simulink model "GraneBaseModel"  (R2023b)
settings: Solver=ode1  StartTime=0.0  StopTime=10  FixedStep=0.01  RelTol=1e-3
undefined symbols (not defined in the file or in its folder): DiscIntNeverNeededParam, National_Instruments, PCI
libraries: sldrtlib x4, simulink x2
settings Model: Creator=labadmin  LastModifiedBy=labadmin
settings SolverCC: AlgebraicLoopSolver=TrustRegion
settings DataIOCC: ReturnWorkspaceOutputs=off
settings DebuggingCC: UnconnectedInputMsg=warning  UnconnectedOutputMsg=warning  UnconnectedLineMsg=warning  ArithmeticOperatorsInVariantConditions=warning
settings HardwareCC: ProdBitPerLong=64  ProdHWDeviceType=Intel->x86-64 (Linux 64)
settings ModelReferenceCC: EnableRefExpFcnMdlSchedulingChecks=on
settings SFSimCC: SimUseLocalCustomCode=off  CustomCodeUndefinedFunction=UseInterfaceOnly
settings RTWCC: Description=Simulink Desktop Real-Time  SystemTargetFile=sldrt.tlc  TemplateMakefile=sldrt.tmf  RTWUseLocalCustomCode=off  RTWCompilerOptimization=on
settings CodeAppCC: MaxIdLength=95
settings SimulinkDesktopRealTimeCC: TargetLibSuffix=_sldrt.a  TargetPreCompLibLocation=C:\Program Files\MATLAB\R2023b\toolbox\sldrt\lib\win64

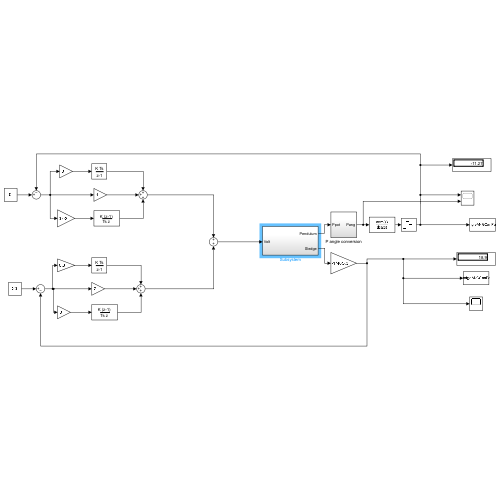
[thumbnail: Simulink's stored preview of the top-level diagram]
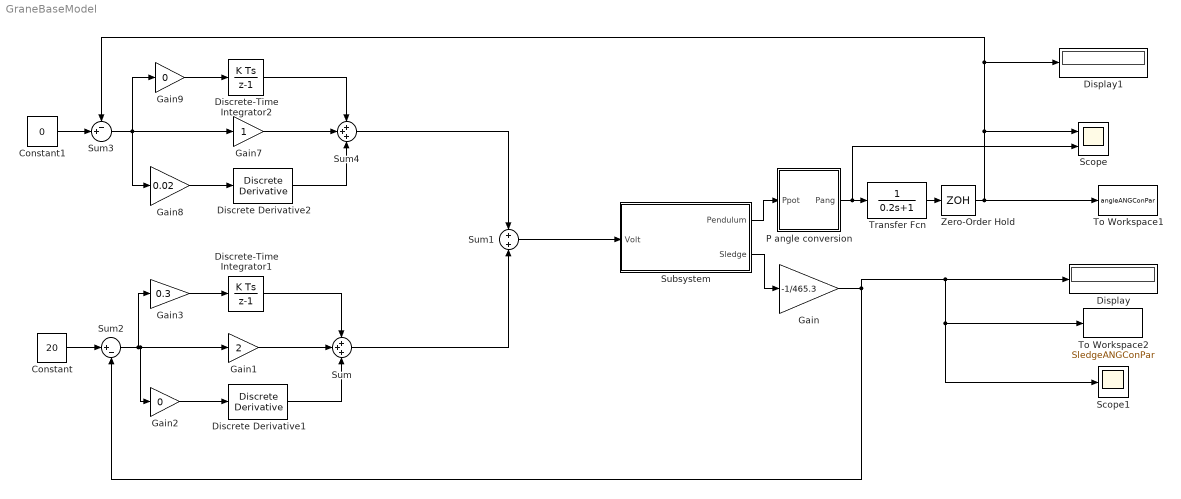
== system GraneBaseModel ==
  Constant : Constant  Value=20
  Constant1 : Constant  Value=0
  Discrete Derivative1 : simulink/Discrete/Discrete Derivative  gainval=1.0  ICPrevScaledInput=0.0  OutMin=[]  OutMax=[]  OutDataType=fixdt(1, 16)  OutScaling=2^-10  DoSatur=off
  Discrete Derivative2 : simulink/Discrete/Discrete Derivative  gainval=1.0  ICPrevScaledInput=0.0  OutMin=[]  OutMax=[]  OutDataType=fixdt(1, 16)  OutScaling=2^-10  DoSatur=off
  Discrete-Time Integrator1 : DiscreteIntegrator  SampleTime=-1  ICPrevOutput=DiscIntNeverNeededParam  ICPrevScaledInput=DiscIntNeverNeededParam
  Discrete-Time Integrator2 : DiscreteIntegrator  SampleTime=-1  ICPrevOutput=DiscIntNeverNeededParam  ICPrevScaledInput=DiscIntNeverNeededParam
  Display : Display
  Display1 : Display
  Gain : Gain  Gain=-1/465.3
  Gain1 : Gain  Gain=2
  Gain2 : Gain  Gain=0
  Gain3 : Gain  Gain=0.3
  Gain7 : Gain
  Gain8 : Gain  Gain=0.02
  Gain9 : Gain  Gain=0
  P angle conversion : Subsystem
  Scope : Scope  NumInputPorts=2
  Scope1 : Scope
  Subsystem : Subsystem
  Sum : Sum  Inputs=+++
  Sum1 : Sum
  Sum2 : Sum  Inputs=|+-
  Sum3 : Sum  Inputs=-+|
  Sum4 : Sum  Inputs=+++
  To Workspace1 : ToWorkspace  VariableName=angleANGConPar  SaveFormat=Timeseries  SampleTime=-1
  To Workspace2 : ToWorkspace  VariableName=SledgeANGConPar  SaveFormat=Timeseries  SampleTime=-1
  Transfer Fcn : TransferFcn  Denominator=[0.2 1]
  Zero-Order Hold : ZeroOrderHold  SampleTime=-1
  wires:
  Subsystem/2(Sledge) -> Gain/1
  Subsystem/1(Pendulum) -> P angle conversion/1(Ppot)
  Gain/1 -> To Workspace2/1, Scope1/1, Display/1, Sum2/2
  Gain1/1 -> Sum/2
  Discrete Derivative1/1 -> Sum/3
  Gain3/1 -> Discrete-Time Integrator1/1
  Gain2/1 -> Discrete Derivative1/1
  Constant/1 -> Sum2/1
  Sum2/1 -> Gain3/1, Gain2/1, Gain1/1
  Discrete-Time Integrator1/1 -> Sum/1
  P angle conversion/1(Pang) -> Scope/2, Transfer Fcn/1
  Zero-Order Hold/1 -> Sum3/1, Display1/1, Scope/1, To Workspace1/1
  Transfer Fcn/1 -> Zero-Order Hold/1
  Gain9/1 -> Discrete-Time Integrator2/1
  Discrete Derivative2/1 -> Sum4/3
  Gain7/1 -> Sum4/2
  Discrete-Time Integrator2/1 -> Sum4/1
  Gain8/1 -> Discrete Derivative2/1
  Sum4/1 -> Sum1/1
  Sum/1 -> Sum1/2
  Constant1/1 -> Sum3/2
  Sum3/1 -> Gain8/1, Gain7/1, Gain9/1
  Sum1/1 -> Subsystem/1(Volt)

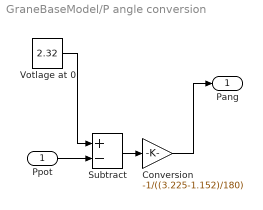
== system GraneBaseModel/P angle conversion ==
  Ppot : Inport
  Conversion : Gain  Gain=-1/((3.225-1.152)/180)
  Subtract : Sum  Inputs=+-
  "Votlage at 0 " : Constant  Value=2.32
  Pang : Outport  VectorParamsAs1DForOutWhenUnconnected=off
  wires:
  Subtract/1 -> Conversion/1
  Ppot/1 -> Subtract/2
  "Votlage at 0 "/1 -> Subtract/1
  Conversion/1 -> Pang/1

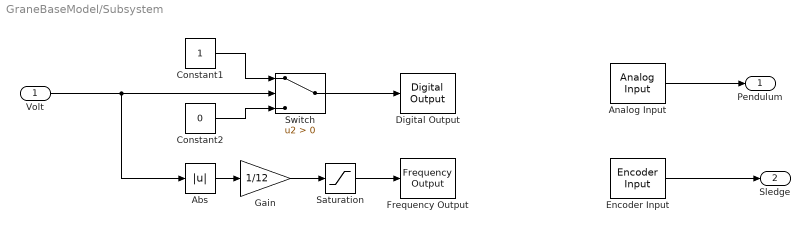
== system GraneBaseModel/Subsystem ==
  Volt : Inport
  Abs : Abs  SaturateOnIntegerOverflow=off
  Analog Input : sldrtlib/Analog Input  SampleTime=-1  MaxMissedTicks=1000000000  ShowMissedTicks=off  YieldWhenWaiting=off  DrvName=National_Instruments/PCI-6229  DrvAddress=4294967295  DrvOptions=[0 1 8192 2 3]  Channels=1  RangeMode=1  VoltRange=1  DataType=1
      settings: AttributesFormatString=National Instruments\nPCI-6229 [auto]
  Constant1 : Constant
  Constant2 : Constant  Value=0
  Digital Output : sldrtlib/Digital Output  SampleTime=-1  MaxMissedTicks=100000000  ShowMissedTicks=off  YieldWhenWaiting=off  DrvName=National_Instruments/PCI-6229  DrvAddress=4294967295  DrvOptions=[0 1 8192 2 3]  Channels=1  BitMode=1  InitialValue=[]  FinalValue=[]
      settings: AttributesFormatString=National Instruments\nPCI-6229 [auto]
  Encoder Input : sldrtlib/Encoder Input  SampleTime=-1  MaxMissedTicks=10000000  ShowMissedTicks=off  YieldWhenWaiting=off  DrvName=National_Instruments/PCI-6229  DrvAddress=4294967295  DrvOptions=[0 1 8192 2 3]  Channels=1  QuadMode=3  IndexPulse=2  InputFilter=Inf  DataType=1
      settings: AttributesFormatString=National Instruments\nPCI-6229 [auto]
  Frequency Output : sldrtlib/Frequency Output  SampleTime=-1  MaxMissedTicks=1000000000  ShowMissedTicks=off  YieldWhenWaiting=off  DrvName=National_Instruments/PCI-6229  DrvAddress=4294967295  DrvOptions=[0 1 8192 2 3]  Channels=2  FrequencySource=1  Frequency=10000  FrequencyFinalValue=[]  DutySource=2  Duty=0  DutyFinalValue=0
      settings: AttributesFormatString=National Instruments\nPCI-6229 [auto]
  Gain : Gain  Gain=1/12
  Saturation : Saturate  UpperLimit=0.35  LowerLimit=0
  Switch : Switch  Criteria=u2 > Threshold  SaturateOnIntegerOverflow=off  InputSameDT=off
  Pendulum : Outport  VectorParamsAs1DForOutWhenUnconnected=off
  Sledge : Outport  Port=2  VectorParamsAs1DForOutWhenUnconnected=off
  wires:
  Analog Input/1 -> Pendulum/1
  Encoder Input/1 -> Sledge/1
  Saturation/1 -> Frequency Output/1
  Volt/1 -> Abs/1, Switch/2
  Gain/1 -> Saturation/1
  Constant2/1 -> Switch/3
  Abs/1 -> Gain/1
  Constant1/1 -> Switch/1
  Switch/1 -> Digital Output/1
